simulink library "sailbot_library"  (R2019a)
settings: Solver=VariableStepAuto  StartTime=0.0  StopTime=10.0  RelTol=1e-3
undefined symbols (not defined in the file or in its folder): A_k, A_r, a_right, A_s, added_mass, b_right, c_heel, d_yaw, I_xx, I_xz, I_zz, k_drag, k_lift, k_rh, m, M, rho_a, rho_w, vss, x_h, x_k, x_m, x_r, x_s, x_sm, X_u_dot, y_h, y_k, y_r, y_s, Y_v_dot, z_h, z_k, z_r, z_s
libraries: $bdroot x16
settings Model: Creator=brucecui  LastModifiedBy=tylerlum
settings DataIOCC: ReturnWorkspaceOutputs=off
settings DebuggingCC: ArithmeticOperatorsInVariantConditions=warning
settings CodeAppCC: StateflowObjectComments=on

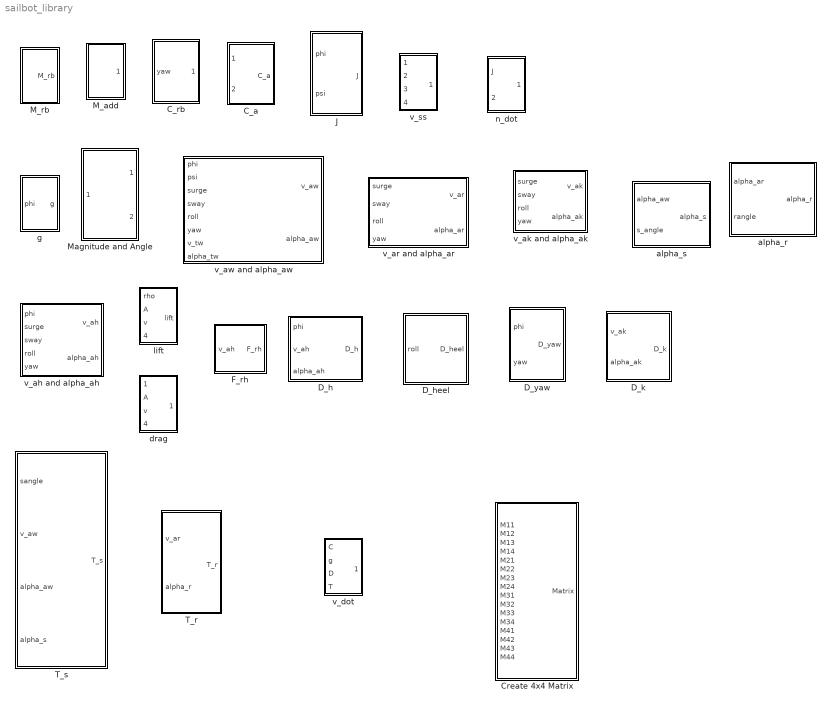
== system sailbot_library ==
  C_a : Subsystem
  C_rb : Subsystem
  Create 4x4 Matrix : Subsystem
  D_h : Subsystem
  "D_heel " : Subsystem
  D_k : Subsystem
  D_yaw : Subsystem
  F_rh : Subsystem
  J : Subsystem
  M_add : Subsystem
  M_rb : Subsystem
  Magnitude and Angle : Subsystem
  T_r : Subsystem
  "T_s " : Subsystem
  alpha_r : Subsystem
  alpha_s : Subsystem
  drag : Subsystem
  g : Subsystem
  lift : Subsystem
  n_dot : Subsystem
  v_ah and alpha_ah : Subsystem
  v_ak and alpha_ak : Subsystem
  v_ar and alpha_ar : Subsystem
  v_aw and alpha_aw : Subsystem
  v_dot : Subsystem
  v_ss : Subsystem

== system sailbot_library/C_a ==
  surge : Inport
  sway : Inport  Port=2
  Constant2 : Constant  Value=0
  Create 4x4 Matrix : $bdroot/Create 4x4 Matrix  SystemSampleTime=-1
  Gain1 : Gain  Gain=X_u_dot
  Gain2 : Gain  Gain=Y_v_dot
  Gain4 : Gain  Gain=-Y_v_dot
  Gain5 : Gain  Gain=-X_u_dot
  Gain6 : Gain  Gain=added_mass
  C_a : Outport
  wires:
  Create 4x4 Matrix/1 -> Gain6/1
  Gain6/1 -> C_a/1
  sway/1 -> Gain2/1, Gain4/1
  surge/1 -> Gain5/1, Gain1/1
  Constant2/1 -> Create 4x4 Matrix/2, Create 4x4 Matrix/1, Create 4x4 Matrix/3, Create 4x4 Matrix/5, Create 4x4 Matrix/6, Create 4x4 Matrix/7, Create 4x4 Matrix/9, Create 4x4 Matrix/10, Create 4x4 Matrix/11, Create 4x4 Matrix/12, Create 4x4 Matrix/15, Create 4x4 Matrix/16
  Gain4/1 -> Create 4x4 Matrix/13
  Gain5/1 -> Create 4x4 Matrix/8
  Gain1/1 -> Create 4x4 Matrix/14
  Gain2/1 -> Create 4x4 Matrix/4

== system sailbot_library/C_rb ==
  yaw : Inport
  Constant1 : Constant  Value=0
  Create 4x4 Matrix1 : $bdroot/Create 4x4 Matrix  SystemSampleTime=-1
  Gain : Gain  Gain=m
  Gain3 : Gain  Gain=-m
  C_rb : Outport
  wires:
  yaw/1 -> Gain3/1, Gain/1
  Create 4x4 Matrix1/1 -> C_rb/1
  Gain/1 -> Create 4x4 Matrix1/5
  Gain3/1 -> Create 4x4 Matrix1/2
  Constant1/1 -> Create 4x4 Matrix1/16, Create 4x4 Matrix1/15, Create 4x4 Matrix1/14, Create 4x4 Matrix1/13, Create 4x4 Matrix1/12, Create 4x4 Matrix1/11, Create 4x4 Matrix1/10, Create 4x4 Matrix1/9, Create 4x4 Matrix1/8, Create 4x4 Matrix1/7, Create 4x4 Matrix1/6, Create 4x4 Matrix1/4, Create 4x4 Matrix1/3, Create 4x4 Matrix1/1

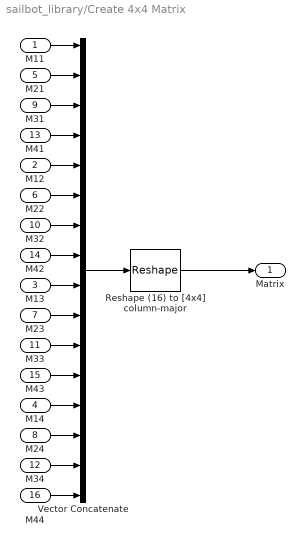
== system sailbot_library/Create 4x4 Matrix ==
  M11 : Inport  PortDimensions=1
  M12 : Inport  Port=2  PortDimensions=1
  M13 : Inport  Port=3  PortDimensions=1
  M14 : Inport  Port=4  PortDimensions=1
  M21 : Inport  Port=5  PortDimensions=1
  M22 : Inport  Port=6  PortDimensions=1
  M23 : Inport  Port=7  PortDimensions=1
  M24 : Inport  Port=8  PortDimensions=1
  M31 : Inport  Port=9  PortDimensions=1
  M32 : Inport  Port=10  PortDimensions=1
  M33 : Inport  Port=11  PortDimensions=1
  M34 : Inport  Port=12  PortDimensions=1
  M41 : Inport  Port=13  PortDimensions=1
  M42 : Inport  Port=14  PortDimensions=1
  M43 : Inport  Port=15  PortDimensions=1
  "M44 " : Inport  Port=16  PortDimensions=1
  Reshape (16) to [4x4] column-major : Reshape  OutputDimensionality=Customize  OutputDimensions=[4,4]
  Vector Concatenate : Concatenate  NumInputs=16
  Matrix : Outport
  wires:
  Reshape (16) to [4x4] column-major/1 -> Matrix/1
  M32/1 -> Vector Concatenate/7
  M13/1 -> Vector Concatenate/9
  M43/1 -> Vector Concatenate/12
  M14/1 -> Vector Concatenate/13
  M11/1 -> Vector Concatenate/1
  M34/1 -> Vector Concatenate/15
  M22/1 -> Vector Concatenate/6
  "M44 "/1 -> Vector Concatenate/16
  M12/1 -> Vector Concatenate/5
  M21/1 -> Vector Concatenate/2
  M24/1 -> Vector Concatenate/14
  Vector Concatenate/1 -> Reshape (16) to [4x4] column-major/1
  M31/1 -> Vector Concatenate/3
  M33/1 -> Vector Concatenate/11
  M42/1 -> Vector Concatenate/8
  M23/1 -> Vector Concatenate/10
  M41/1 -> Vector Concatenate/4

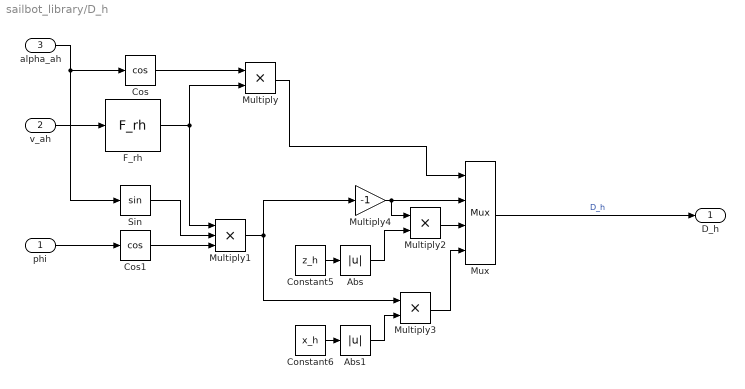
== system sailbot_library/D_h ==
  phi : Inport
  v_ah : Inport  Port=2
  alpha_ah : Inport  Port=3
  Abs : Abs
  Abs1 : Abs
  Constant5 : Constant  Value=z_h
  Constant6 : Constant  Value=x_h
  Cos : Trigonometry  Operator=cos
  Cos1 : Trigonometry  Operator=cos
  F_rh : $bdroot/F_rh  SystemSampleTime=-1
  Multiply : Product
  Multiply1 : Product  Inputs=3
  Multiply2 : Product
  Multiply3 : Product
  Multiply4 : Gain  Gain=-1
  Mux : Mux
  Sin : Trigonometry
  D_h : Outport
  wires:
  phi/1 -> Cos1/1
  Sin/1 -> Multiply1/2
  v_ah/1 -> F_rh/1
  Multiply/1 -> Mux/1
  Mux/1 -> D_h/1  "D_h"
  Cos/1 -> Multiply/1
  F_rh/1 -> Multiply1/1, Multiply/2
  alpha_ah/1 -> Sin/1, Cos/1
  Multiply3/1 -> Mux/4
  Multiply1/1 -> Multiply4/1, Multiply3/1
  Multiply2/1 -> Mux/3
  Multiply4/1 -> Multiply2/1, Mux/2
  Cos1/1 -> Multiply1/3
  Constant5/1 -> Abs/1
  Abs/1 -> Multiply2/2
  Constant6/1 -> Abs1/1
  Abs1/1 -> Multiply3/2

== system sailbot_library/D_heel  ==
  roll : Inport
  Abs : Abs
  Constant5 : Constant  Value=0
  Gain : Gain  Gain=c_heel
  Multiply : Product
  Mux : Mux
  D_heel : Outport
  wires:
  Multiply/1 -> Mux/3
  Gain/1 -> Multiply/1
  Constant5/1 -> Mux/1, Mux/2, Mux/4
  Mux/1 -> D_heel/1  "D_heel"
  Abs/1 -> Multiply/2
  roll/1 -> Abs/1, Gain/1

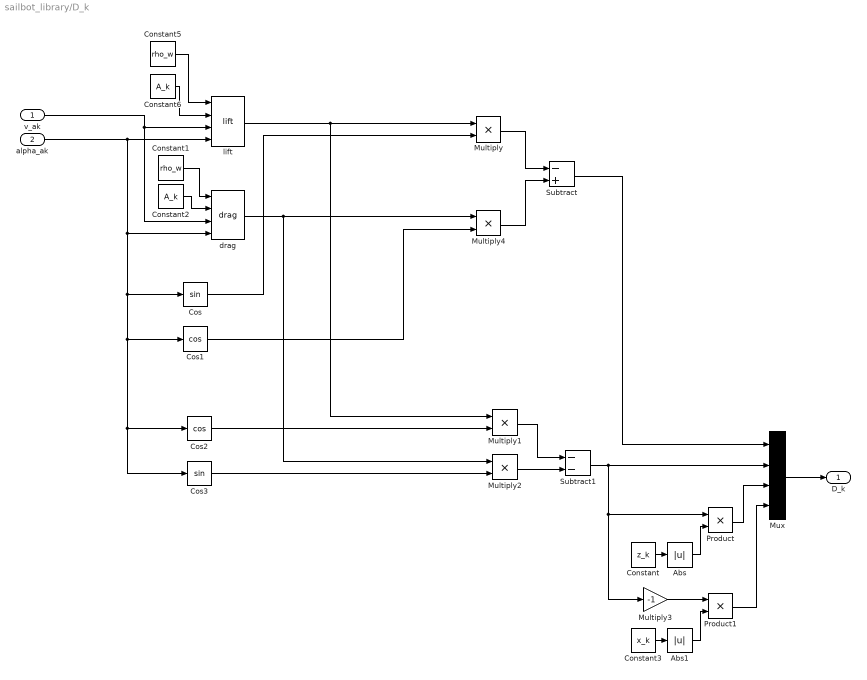
== system sailbot_library/D_k ==
  v_ak : Inport
  alpha_ak : Inport  Port=2
  Abs : Abs
  Abs1 : Abs
  Constant : Constant  Value=z_k
  Constant1 : Constant  Value=rho_w
  Constant2 : Constant  Value=A_k
  Constant3 : Constant  Value=x_k
  Constant5 : Constant  Value=rho_w
  Constant6 : Constant  Value=A_k
  Cos : Trigonometry
  Cos1 : Trigonometry  Operator=cos
  Cos2 : Trigonometry  Operator=cos
  Cos3 : Trigonometry
  Multiply{,1..2,4} (4 alike) : Product
  Multiply3 : Gain  Gain=-1
  Mux : Mux
  Product : Product
  Product1 : Product
  Subtract : Sum  Inputs=-+
  Subtract1 : Sum  Inputs=--
  drag : $bdroot/drag  SystemSampleTime=-1
  lift : $bdroot/lift  SystemSampleTime=-1
  D_k : Outport
  wires:
  Abs/1 -> Product/2
  Constant3/1 -> Abs1/1
  Cos1/1 -> Multiply4/2
  Mux/1 -> D_k/1
  lift/1 -> Multiply1/1, Multiply/1
  Multiply1/1 -> Subtract1/1
  Constant1/1 -> drag/1
  Cos/1 -> Multiply/2
  Constant/1 -> Abs/1
  Multiply4/1 -> Subtract/2
  Abs1/1 -> Product1/2
  Subtract1/1 -> Product/1, Multiply3/1, Mux/2
  Constant2/1 -> drag/2
  Product/1 -> Mux/3
  alpha_ak/1 -> drag/4, Cos2/1, Cos3/1, Cos1/1, Cos/1, lift/4
  drag/1 -> Multiply2/1, Multiply4/1
  Cos3/1 -> Multiply2/2
  Subtract/1 -> Mux/1
  Product1/1 -> Mux/4
  Multiply3/1 -> Product1/1
  Multiply/1 -> Subtract/1
  v_ak/1 -> lift/3, drag/3
  Constant6/1 -> lift/2
  Cos2/1 -> Multiply1/2
  Multiply2/1 -> Subtract1/2
  Constant5/1 -> lift/1

== system sailbot_library/D_yaw ==
  phi : Inport
  yaw : Inport  Port=2
  Abs : Abs
  Constant5 : Constant  Value=0
  Cos : Trigonometry  Operator=cos
  Gain : Gain  Gain=d_yaw
  Multiply : Product  Inputs=3
  Mux : Mux
  Product : Product
  D_yaw : Outport
  wires:
  Constant5/1 -> Mux/1, Mux/2, Mux/3
  Abs/1 -> Multiply/2
  phi/1 -> Cos/1
  Multiply/1 -> Mux/4
  Cos/1 -> Multiply/3, Product/2
  Gain/1 -> Multiply/1
  Mux/1 -> D_yaw/1  "D_yaw"
  Product/1 -> Gain/1, Abs/1
  yaw/1 -> Product/1

== system sailbot_library/F_rh ==
  v_ah : Inport
  Multiply : Gain  Gain=k_rh
  Square : Math  Operator=square  SaturateOnIntegerOverflow=on
  F_rh : Outport
  wires:
  v_ah/1 -> Square/1
  Square/1 -> Multiply/1
  Multiply/1 -> F_rh/1

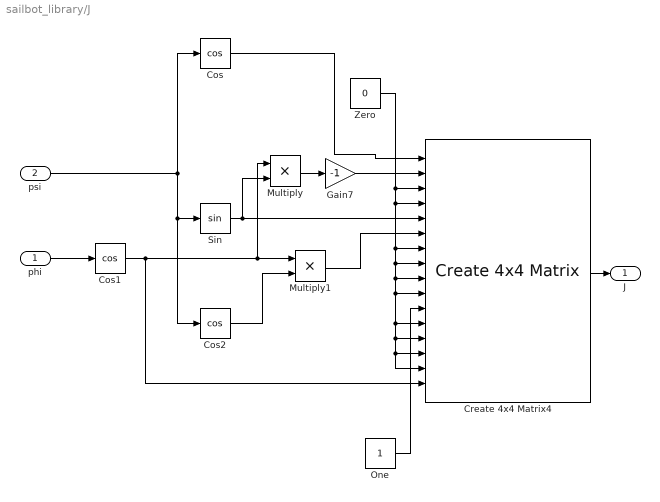
== system sailbot_library/J ==
  phi : Inport
  psi : Inport  Port=2
  Cos : Trigonometry  Operator=cos
  Cos1 : Trigonometry  Operator=cos
  Cos2 : Trigonometry  Operator=cos
  Create 4x4 Matrix4 : $bdroot/Create 4x4 Matrix  SystemSampleTime=-1
  Gain7 : Gain  Gain=-1
  Multiply : Product
  Multiply1 : Product
  One : Constant  OutDataTypeStr=Inherit: Inherit via back propagation
  Sin : Trigonometry
  Zero : Constant  Value=0  OutDataTypeStr=Inherit: Inherit via back propagation
  J : Outport
  wires:
  phi/1 -> Cos1/1
  One/1 -> Create 4x4 Matrix4/11
  Sin/1 -> Multiply/2, Create 4x4 Matrix4/5
  Cos2/1 -> Multiply1/2
  Create 4x4 Matrix4/1 -> J/1
  Cos/1 -> Create 4x4 Matrix4/1
  Cos1/1 -> Multiply/1, Multiply1/1, Create 4x4 Matrix4/16
  psi/1 -> Cos2/1, Sin/1, Cos/1
  Multiply1/1 -> Create 4x4 Matrix4/6
  Gain7/1 -> Create 4x4 Matrix4/2
  Multiply/1 -> Gain7/1
  Zero/1 -> Create 4x4 Matrix4/3, Create 4x4 Matrix4/4, Create 4x4 Matrix4/8, Create 4x4 Matrix4/9, Create 4x4 Matrix4/10, Create 4x4 Matrix4/12, Create 4x4 Matrix4/13, Create 4x4 Matrix4/14, Create 4x4 Matrix4/15, Create 4x4 Matrix4/7

== system sailbot_library/M_add ==
  Constant4 : Constant  Value=0
  Constant5 : Constant  Value=added_mass
  Create 4x4 Matrix3 : $bdroot/Create 4x4 Matrix  SystemSampleTime=-1
  M_add : Outport
  wires:
  Constant4/1 -> Create 4x4 Matrix3/3, Create 4x4 Matrix3/2, Create 4x4 Matrix3/4, Create 4x4 Matrix3/5, Create 4x4 Matrix3/7, Create 4x4 Matrix3/14, Create 4x4 Matrix3/15, Create 4x4 Matrix3/13, Create 4x4 Matrix3/12, Create 4x4 Matrix3/10, Create 4x4 Matrix3/9, Create 4x4 Matrix3/8
  Create 4x4 Matrix3/1 -> M_add/1
  Constant5/1 -> Create 4x4 Matrix3/1, Create 4x4 Matrix3/11, Create 4x4 Matrix3/16, Create 4x4 Matrix3/6

== system sailbot_library/M_rb ==
  -I_xz : Constant  Value=-I_xz
  Constant3 : Constant  Value=0
  Create 4x4 Matrix2 : $bdroot/Create 4x4 Matrix  SystemSampleTime=-1
  I_xx : Constant  Value=I_xx
  I_xz : Constant  Value=I_xz
  I_zz : Constant  Value=I_zz
  m : Constant  Value=m
  M_rb : Outport
  wires:
  m/1 -> Create 4x4 Matrix2/6, Create 4x4 Matrix2/1
  Create 4x4 Matrix2/1 -> M_rb/1
  Constant3/1 -> Create 4x4 Matrix2/14, Create 4x4 Matrix2/13, Create 4x4 Matrix2/10, Create 4x4 Matrix2/9, Create 4x4 Matrix2/8, Create 4x4 Matrix2/7, Create 4x4 Matrix2/5, Create 4x4 Matrix2/4, Create 4x4 Matrix2/3, Create 4x4 Matrix2/2
  -I_xz/1 -> Create 4x4 Matrix2/15
  I_zz/1 -> Create 4x4 Matrix2/16
  I_xz/1 -> Create 4x4 Matrix2/12
  I_xx/1 -> Create 4x4 Matrix2/11

== system sailbot_library/Magnitude and Angle ==
  Vector : Inport
  Atan2 : Trigonometry  Operator=atan2
  Demux : Demux  Outputs=2
  Dot Product : DotProduct  InputSameDT=on  OutDataTypeStr=Inherit: Inherit via internal rule
  Gain : Gain  Gain=-1
  Sqrt : Sqrt  SaturateOnIntegerOverflow=on
  Magnitude : Outport
  Angle : Outport  Port=2
  wires:
  Dot Product/1 -> Sqrt/1
  Sqrt/1 -> Magnitude/1
  Atan2/1 -> Angle/1
  Demux/2 -> Atan2/1
  Vector/1 -> Dot Product/1, Dot Product/2, Demux/1
  Gain/1 -> Atan2/2
  Demux/1 -> Gain/1

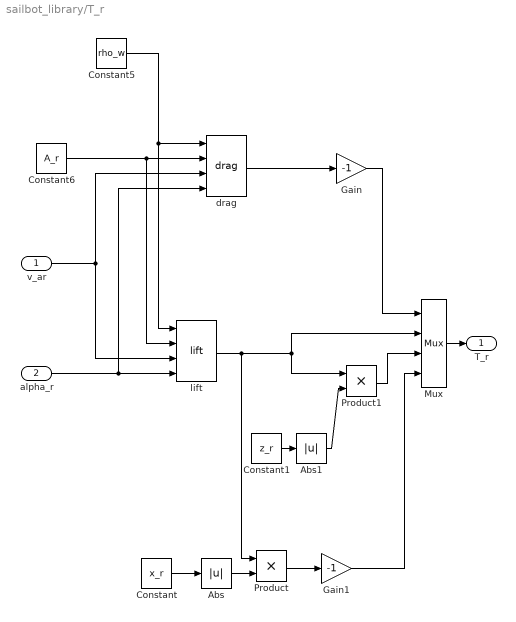
== system sailbot_library/T_r ==
  v_ar : Inport
  alpha_r : Inport  Port=2
  Abs : Abs
  Abs1 : Abs
  Constant : Constant  Value=x_r
  Constant1 : Constant  Value=z_r
  Constant5 : Constant  Value=rho_w
  Constant6 : Constant  Value=A_r
  Gain : Gain  Gain=-1
  Gain1 : Gain  Gain=-1
  Mux : Mux
  Product : Product
  Product1 : Product
  drag : $bdroot/drag  SystemSampleTime=-1
  lift : $bdroot/lift  SystemSampleTime=-1
  T_r : Outport
  wires:
  Mux/1 -> T_r/1
  Constant5/1 -> lift/1, drag/1
  lift/1 -> Product/1, Product1/1, Mux/2
  Product1/1 -> Mux/3
  alpha_r/1 -> drag/4, lift/4
  v_ar/1 -> lift/3, drag/3
  Constant6/1 -> lift/2, drag/2
  Gain/1 -> Mux/1
  drag/1 -> Gain/1
  Constant/1 -> Abs/1
  Abs/1 -> Product/2
  Constant1/1 -> Abs1/1
  Abs1/1 -> Product1/2
  Product/1 -> Gain1/1
  Gain1/1 -> Mux/4

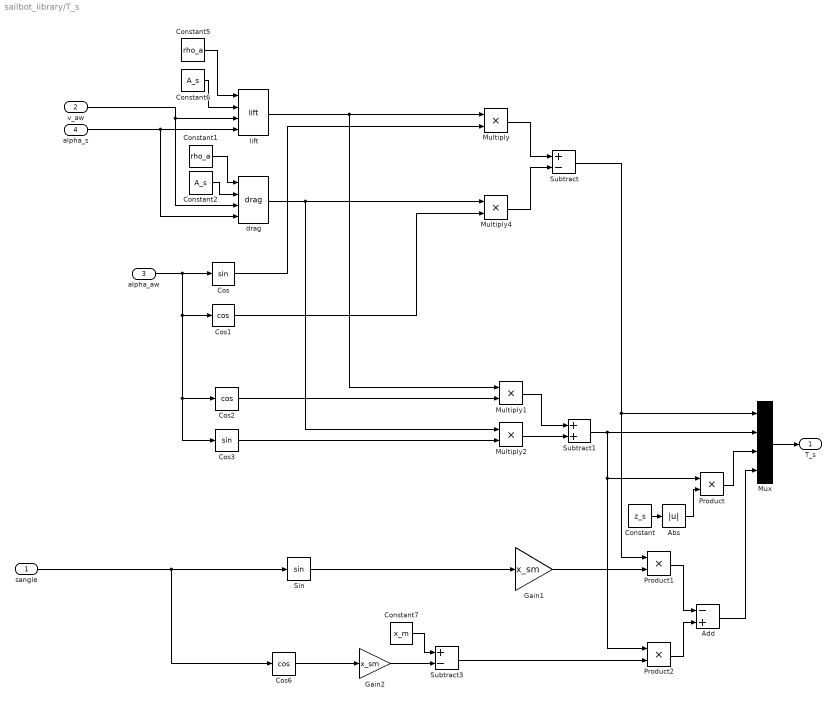
== system sailbot_library/T_s  ==
  sangle : Inport
  v_aw : Inport  Port=2
  alpha_aw : Inport  Port=3
  alpha_s : Inport  Port=4
  Abs : Abs
  Add : Sum  Inputs=-+
  Constant : Constant  Value=z_s
  Constant1 : Constant  Value=rho_a
  Constant2 : Constant  Value=A_s
  Constant5 : Constant  Value=rho_a
  Constant6 : Constant  Value=A_s
  Constant7 : Constant  Value=x_m
  Cos : Trigonometry
  Cos1 : Trigonometry  Operator=cos
  Cos2 : Trigonometry  Operator=cos
  Cos3 : Trigonometry
  Cos6 : Trigonometry  Operator=cos
  Gain1 : Gain  Gain=x_sm
  Gain2 : Gain  Gain=x_sm
  Multiply{,1..2,4} (4 alike) : Product
  Mux : Mux
  Product : Product
  Product1 : Product
  Product2 : Product
  Sin : Trigonometry
  Subtract : Sum  Inputs=+-
  Subtract1 : Sum
  Subtract3 : Sum  Inputs=+-
  drag : $bdroot/drag  SystemSampleTime=-1
  lift : $bdroot/lift  SystemSampleTime=-1
  T_s : Outport
  wires:
  sangle/1 -> Cos6/1, Sin/1
  Constant7/1 -> Subtract3/1
  lift/1 -> Multiply1/1, Multiply/1
  alpha_aw/1 -> Cos1/1, Cos3/1, Cos2/1, Cos/1
  alpha_s/1 -> drag/4, lift/4
  Multiply2/1 -> Subtract1/2
  v_aw/1 -> lift/3, drag/3
  Constant1/1 -> drag/1
  Constant2/1 -> drag/2
  Mux/1 -> T_s/1
  Cos/1 -> Multiply/2
  Multiply1/1 -> Subtract1/1
  drag/1 -> Multiply2/1, Multiply4/1
  Constant6/1 -> lift/2
  Cos3/1 -> Multiply2/2
  Constant5/1 -> lift/1
  Cos1/1 -> Multiply4/2
  Subtract3/1 -> Product2/2
  Gain2/1 -> Subtract3/2
  Cos2/1 -> Multiply1/2
  Subtract1/1 -> Product/1, Product2/1, Mux/2
  Multiply4/1 -> Subtract/2
  Multiply/1 -> Subtract/1
  Cos6/1 -> Gain2/1
  Subtract/1 -> Product1/1, Mux/1
  Sin/1 -> Gain1/1
  Constant/1 -> Abs/1
  Abs/1 -> Product/2
  Product/1 -> Mux/3
  Add/1 -> Mux/4
  Product2/1 -> Add/2
  Product1/1 -> Add/1
  Gain1/1 -> Product1/2

== system sailbot_library/alpha_r ==
  alpha_ar : Inport
  rangle : Inport  Port=2
  Add : Sum  Inputs=+-
  alpha_r : Outport
  wires:
  Add/1 -> alpha_r/1
  rangle/1 -> Add/2
  alpha_ar/1 -> Add/1

== system sailbot_library/alpha_s ==
  alpha_aw : Inport
  s_angle : Inport  Port=2
  Add : Sum  Inputs=+-
  alpha_s : Outport
  wires:
  alpha_aw/1 -> Add/1
  s_angle/1 -> Add/2
  Add/1 -> alpha_s/1

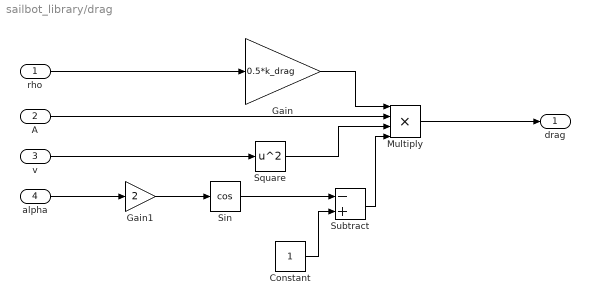
== system sailbot_library/drag ==
  rho : Inport
  A : Inport  Port=2
  v : Inport  Port=3
  alpha : Inport  Port=4
  Constant : Constant
  Gain : Gain  Gain=0.5*k_drag
  Gain1 : Gain  Gain=2
  Multiply : Product  Inputs=4
  Sin : Trigonometry  Operator=cos
  Square : Math  Operator=square  SaturateOnIntegerOverflow=on
  Subtract : Sum  Inputs=-+
  drag : Outport
  wires:
  rho/1 -> Gain/1
  alpha/1 -> Gain1/1
  Gain/1 -> Multiply/1
  v/1 -> Square/1
  A/1 -> Multiply/2
  Square/1 -> Multiply/3
  Gain1/1 -> Sin/1
  Multiply/1 -> drag/1
  Subtract/1 -> Multiply/4
  Sin/1 -> Subtract/1
  Constant/1 -> Subtract/2

== system sailbot_library/g ==
  phi : Inport
  Add1 : Sum
  Constant : Constant  Value=a_right
  Constant6 : Constant  Value=0
  Constant7 : Constant  Value=b_right
  Math Function : Math  Operator=square  SaturateOnIntegerOverflow=on
  Mux3 : Mux
  Product : Product
  Product1 : Product
  g : Outport
  wires:
  phi/1 -> Product1/1, Math Function/1
  Product1/1 -> Add1/2
  Product/1 -> Add1/1
  Add1/1 -> Mux3/3
  Constant/1 -> Product/1
  Math Function/1 -> Product/2
  Constant7/1 -> Product1/2
  Constant6/1 -> Mux3/4, Mux3/2, Mux3/1
  Mux3/1 -> g/1

== system sailbot_library/lift ==
  rho : Inport
  A : Inport  Port=2
  v : Inport  Port=3
  alpha : Inport  Port=4
  Gain : Gain  Gain=0.5*k_lift
  Gain1 : Gain  Gain=2
  Multiply : Product  Inputs=4
  Sin : Trigonometry
  Square : Math  Operator=square  SaturateOnIntegerOverflow=on
  lift : Outport
  wires:
  rho/1 -> Gain/1
  alpha/1 -> Gain1/1
  Gain/1 -> Multiply/1
  Sin/1 -> Multiply/4
  v/1 -> Square/1
  A/1 -> Multiply/2
  Square/1 -> Multiply/3
  Gain1/1 -> Sin/1
  Multiply/1 -> lift/1

== system sailbot_library/n_dot ==
  J : Inport
  v_ss : Inport  Port=2
  Product12 : Product  Multiplication=Matrix(*)
  n_dot : Outport
  wires:
  J/1 -> Product12/1
  v_ss/1 -> Product12/2
  Product12/1 -> n_dot/1

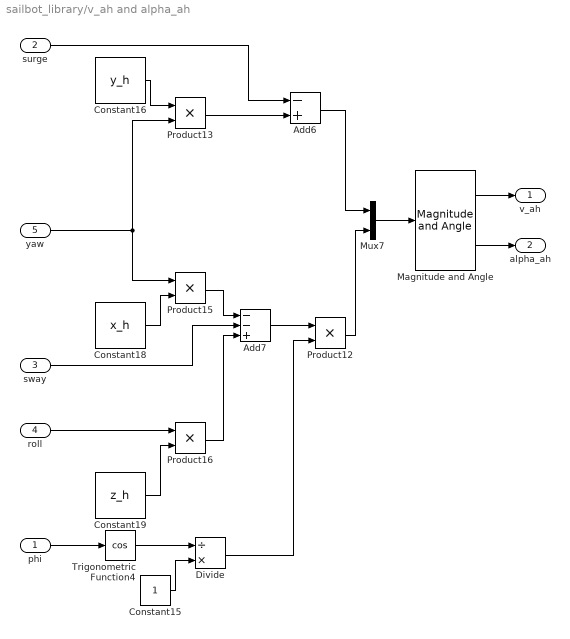
== system sailbot_library/v_ah and alpha_ah ==
  phi : Inport
  "surge " : Inport  Port=2
  sway : Inport  Port=3
  roll : Inport  Port=4
  yaw : Inport  Port=5
  Add6 : Sum  Inputs=-+
  Add7 : Sum  Inputs=--+
  Constant15 : Constant
  Constant16 : Constant  Value=y_h
  Constant18 : Constant  Value=x_h
  Constant19 : Constant  Value=z_h
  Divide : Product  Inputs=/*
  Magnitude and Angle : $bdroot/Magnitude and Angle  SystemSampleTime=-1
  Mux7 : Mux  Inputs=2
  Product{12..13,15..16} (4 alike) : Product
  Trigonometric Function4 : Trigonometry  Operator=cos
  v_ah : Outport
  alpha_ah : Outport  Port=2
  wires:
  sway/1 -> Add7/2
  Product12/1 -> Mux7/2
  Divide/1 -> Product12/2
  Add7/1 -> Product12/1
  Product13/1 -> Add6/2
  Constant18/1 -> Product15/2
  Constant15/1 -> Divide/2
  Constant19/1 -> Product16/2
  yaw/1 -> Product15/1, Product13/2
  "surge "/1 -> Add6/1
  Add6/1 -> Mux7/1
  phi/1 -> Trigonometric Function4/1
  Constant16/1 -> Product13/1
  roll/1 -> Product16/1
  Trigonometric Function4/1 -> Divide/1
  Product15/1 -> Add7/1
  Product16/1 -> Add7/3
  Mux7/1 -> Magnitude and Angle/1
  Magnitude and Angle/1 -> v_ah/1
  Magnitude and Angle/2 -> alpha_ah/1

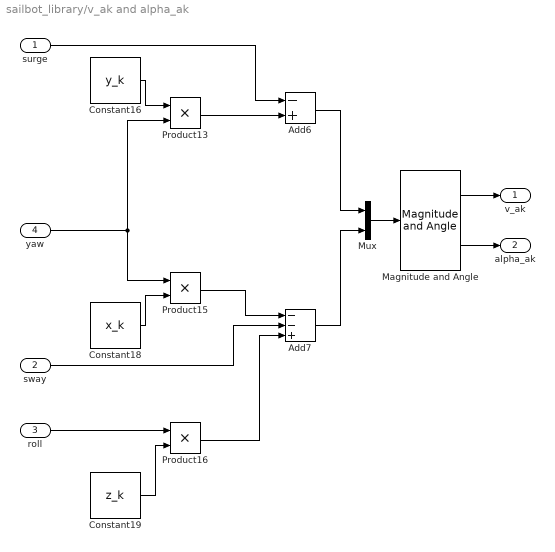
== system sailbot_library/v_ak and alpha_ak ==
  "surge " : Inport
  sway : Inport  Port=2
  roll : Inport  Port=3
  yaw : Inport  Port=4
  Add6 : Sum  Inputs=-+
  Add7 : Sum  Inputs=--+
  Constant16 : Constant  Value=y_k
  Constant18 : Constant  Value=x_k
  Constant19 : Constant  Value=z_k
  Magnitude and Angle : $bdroot/Magnitude and Angle  SystemSampleTime=-1
  Mux : Mux  Inputs=2
  Product13 : Product
  Product15 : Product
  Product16 : Product
  v_ak : Outport
  alpha_ak : Outport  Port=2
  wires:
  Add7/1 -> Mux/2
  Add6/1 -> Mux/1
  Constant18/1 -> Product15/2
  Constant19/1 -> Product16/2
  Product16/1 -> Add7/3
  yaw/1 -> Product13/2, Product15/1
  Constant16/1 -> Product13/1
  roll/1 -> Product16/1
  Product13/1 -> Add6/2
  "surge "/1 -> Add6/1
  Product15/1 -> Add7/1
  sway/1 -> Add7/2
  Mux/1 -> Magnitude and Angle/1
  Magnitude and Angle/1 -> v_ak/1
  Magnitude and Angle/2 -> alpha_ak/1

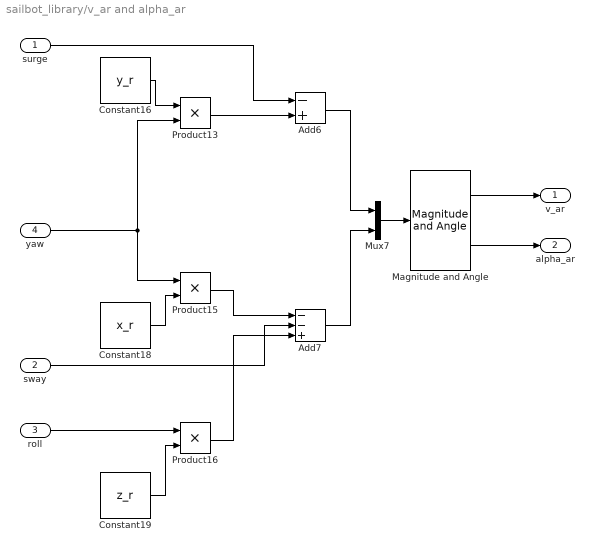
== system sailbot_library/v_ar and alpha_ar ==
  surge : Inport
  sway : Inport  Port=2
  roll : Inport  Port=3
  yaw : Inport  Port=4
  Add6 : Sum  Inputs=-+
  Add7 : Sum  Inputs=--+
  Constant16 : Constant  Value=y_r
  Constant18 : Constant  Value=x_r
  Constant19 : Constant  Value=z_r
  Magnitude and Angle : $bdroot/Magnitude and Angle  SystemSampleTime=-1
  Mux7 : Mux  Inputs=2
  Product13 : Product
  Product15 : Product
  Product16 : Product
  v_ar : Outport
  alpha_ar : Outport  Port=2
  wires:
  Add7/1 -> Mux7/2
  Product15/1 -> Add7/1
  sway/1 -> Add7/2
  yaw/1 -> Product15/1, Product13/2
  Mux7/1 -> Magnitude and Angle/1
  Constant19/1 -> Product16/2
  Constant16/1 -> Product13/1
  roll/1 -> Product16/1
  Constant18/1 -> Product15/2
  Product16/1 -> Add7/3
  Product13/1 -> Add6/2
  surge/1 -> Add6/1
  Add6/1 -> Mux7/1
  Magnitude and Angle/1 -> v_ar/1
  Magnitude and Angle/2 -> alpha_ar/1

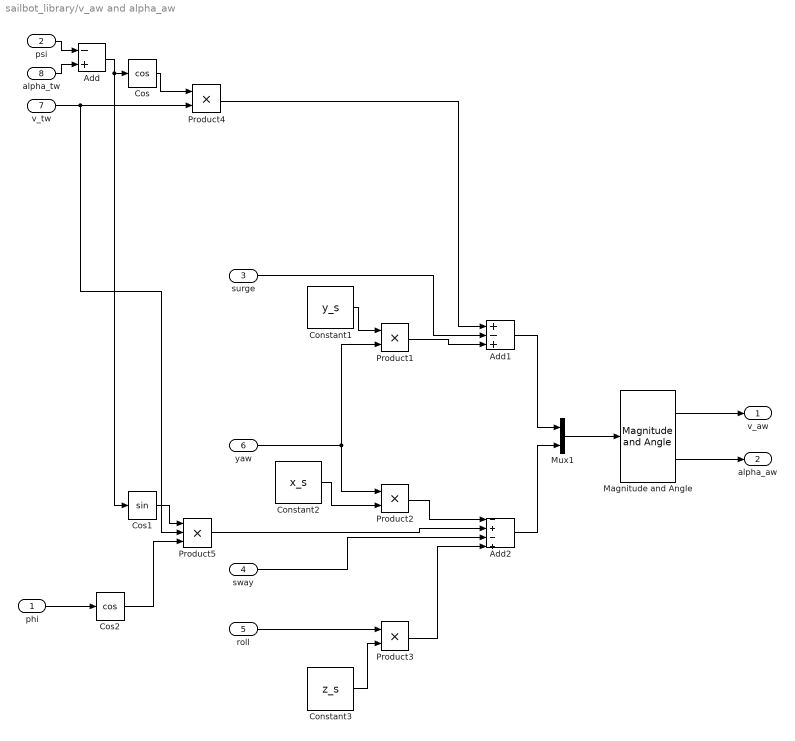
== system sailbot_library/v_aw and alpha_aw ==
  phi : Inport
  psi : Inport  Port=2
  surge : Inport  Port=3
  sway : Inport  Port=4
  roll : Inport  Port=5
  yaw : Inport  Port=6
  v_tw : Inport  Port=7
  alpha_tw : Inport  Port=8
  Add : Sum  Inputs=-+
  Add1 : Sum  Inputs=+-+
  Add2 : Sum  Inputs=-+-+
  Constant1 : Constant  Value=y_s
  Constant2 : Constant  Value=x_s
  Constant3 : Constant  Value=z_s
  Cos : Trigonometry  Operator=cos
  Cos1 : Trigonometry
  Cos2 : Trigonometry  Operator=cos
  Magnitude and Angle : $bdroot/Magnitude and Angle  SystemSampleTime=-1
  Mux1 : Mux  Inputs=2
  Product{1..4} (4 alike) : Product
  Product5 : Product  Inputs=3
  v_aw : Outport
  alpha_aw : Outport  Port=2
  wires:
  Product2/1 -> Add2/1
  sway/1 -> Add2/3
  surge/1 -> Add1/2
  Product3/1 -> Add2/4
  phi/1 -> Cos2/1
  alpha_tw/1 -> Add/2
  Product4/1 -> Add1/1
  psi/1 -> Add/1
  Product1/1 -> Add1/3
  Constant1/1 -> Product1/1
  Add/1 -> Cos/1, Cos1/1
  Constant2/1 -> Product2/2
  Cos2/1 -> Product5/3
  v_tw/1 -> Product4/2, Product5/2
  yaw/1 -> Product2/1, Product1/2
  Add1/1 -> Mux1/1
  Cos1/1 -> Product5/1
  Constant3/1 -> Product3/2
  Add2/1 -> Mux1/2
  Product5/1 -> Add2/2
  roll/1 -> Product3/1
  Cos/1 -> Product4/1
  Mux1/1 -> Magnitude and Angle/1
  Magnitude and Angle/1 -> v_aw/1
  Magnitude and Angle/2 -> alpha_aw/1

== system sailbot_library/v_dot ==
  C : Inport
  g : Inport  Port=2
  D : Inport  Port=3
  T : Inport  Port=4
  Gain : Gain  Gain=-inv(M)  Multiplication=Matrix(K*u)
  Gain1 : Gain  Gain=-inv(M)  Multiplication=Matrix(K*u)
  Gain2 : Gain  Gain=inv(M)  Multiplication=Matrix(K*u)
  Gain3 : Gain  Gain=-inv(M)  Multiplication=Matrix(K*u)
  Gain4 : Gain  Gain=vss  Multiplication=Matrix(u*K)
  Sum : Sum  Inputs=4
  v_dot : Outport
  wires:
  g/1 -> Gain1/1
  T/1 -> Gain2/1
  Gain1/1 -> Sum/3
  D/1 -> Gain3/1
  Gain4/1 -> Gain/1
  Sum/1 -> v_dot/1  "v_dot"
  Gain3/1 -> Sum/2
  Gain/1 -> Sum/1
  Gain2/1 -> Sum/4
  C/1 -> Gain4/1

== system sailbot_library/v_ss ==
  surge : Inport
  sway : Inport  Port=2
  roll : Inport  Port=3
  yaw : Inport  Port=4
  Mux7 : Mux
  v_ss : Outport
  wires:
  sway/1 -> Mux7/2
  surge/1 -> Mux7/1
  yaw/1 -> Mux7/4
  roll/1 -> Mux7/3
  Mux7/1 -> v_ss/1
